simulink model "lvdt"  (R2020a)
settings: Solver=VariableStepAuto  StartTime=0.0  StopTime=120  RelTol=1e-3
settings Model: Creator=Sumit  LastModifiedBy=Sumit
settings SolverCC: ZeroCrossAlgorithm=Adaptive
settings DebuggingCC: IgnoredZcDiagnostic=none

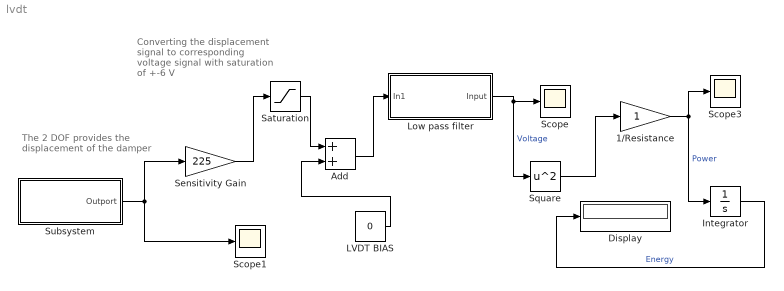
== system lvdt ==
  note: The 2 DOF provides the displacement of the damper
  note: Converting the displacement signal to corresponding voltage signal with saturation of +-6 V
  1/Resistance : Gain
  Add : Sum
  Display : Display
  Integrator : Integrator
  LVDT BIAS : Constant  Value=0
  Low pass filter : Subsystem
  Saturation : Saturate  UpperLimit=6  LowerLimit=-6
  Scope : Scope
  Scope1 : Scope
  Scope3 : Scope
  Sensitivity Gain : Gain  Gain=225
  Square : Math  Operator=square  SaturateOnIntegerOverflow=on
  Subsystem : Subsystem
  wires:
  Sensitivity Gain/1 -> Saturation/1
  Saturation/1 -> Add/1
  LVDT BIAS/1 -> Add/2
  Add/1 -> Low pass filter/1(In1)
  Low pass filter/1(Input) -> Square/1, Scope/1  "Voltage"
  Subsystem/1(Outport) -> Sensitivity Gain/1, Scope1/1
  Square/1 -> 1/Resistance/1
  1/Resistance/1 -> Integrator/1, Scope3/1  "Power"
  Integrator/1 -> Display/1  "Energy"

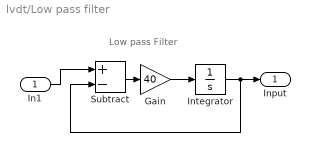
== system lvdt/Low pass filter ==
  note: Low pass Filter
  In1 : Inport
  Gain : Gain  Gain=40
  Integrator : Integrator
  Subtract : Sum  Inputs=+-
  Input : Outport
  wires:
  In1/1 -> Subtract/1
  Subtract/1 -> Gain/1
  Gain/1 -> Integrator/1
  Integrator/1 -> Subtract/2, Input/1

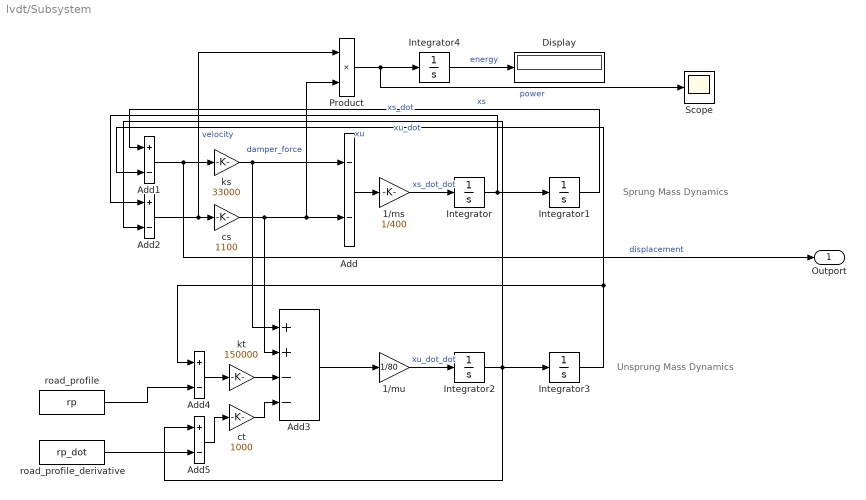
== system lvdt/Subsystem ==
  note: Sprung Mass Dynamics
  note: Unsprung Mass Dynamics
  1/ms : Gain  Gain=1/400
  1/mu : Gain  Gain=1/80
  Add : Sum  Inputs=--
  Add{1..2,4..5} (4 alike) : Sum  Inputs=+-
  Add3 : Sum  Inputs=++--
  Display : Display
      settings: Decimation=2
  Integrator{,1..4} (5 alike) : Integrator
  Product : Product
  Scope : Scope
  cs : Gain  Gain=1100
  ct : Gain  Gain=1000
  ks : Gain  Gain=33000
  kt : Gain  Gain=150000
  road_profile : FromWorkspace  VariableName=rp
  road_profile_derivative : FromWorkspace  VariableName=rp_dot
  Outport : Outport
  wires:
  cs/1 -> Add3/2, Add/2, Product/2  "damper_force"
  Product/1 -> Scope/1, Integrator4/1  "power"
  kt/1 -> Add3/3
  Integrator4/1 -> Display/1  "energy"
  Integrator/1 -> Integrator1/1, Add2/1  "xs_dot"
  Add2/1 -> Product/1, cs/1  "velocity"
  Integrator1/1 -> Add1/1  "xs"
  Add1/1 -> Outport/1, ks/1  "displacement"
  Add/1 -> 1/ms/1
  ct/1 -> Add3/4
  ks/1 -> Add3/1, Add/1
  Add3/1 -> 1/mu/1
  road_profile/1 -> Add4/2
  Integrator3/1 -> Add1/2, Add4/1  "xu"
  Integrator2/1 -> Add5/1, Add2/2, Integrator3/1  "xu_dot"
  Add4/1 -> kt/1
  road_profile_derivative/1 -> Add5/2
  1/mu/1 -> Integrator2/1  "xu_dot_dot"
  1/ms/1 -> Integrator/1  "xs_dot_dot"
  Add5/1 -> ct/1
